simulink library "ET3036TU_model_library_2021b"  (R2021b)
settings: Solver=VariableStepAuto  StartTime=0.0  StopTime=10.0  RelTol=1e-3
values from neighbouring files (symbols this model uses):
  Data =     [Data.mat]
  E_tol = 100    [run_test.m]
  Fnom = 50    [run_test.m]
  OverChargingProtection = 0    [run_test.m]
  simulation_mode = 2    [run_test.m]
  T_err = 60*60    (= 3600)    [run_test.m]
  Tsample = 60    [run_test.m]
  Vnom = sqrt(3)*230    [run_test.m]
undefined symbols (not defined in the file or in its folder): sigbuilder_block, sim_text
libraries: simulink x13, spsThreePhaseDynamicLoadLib x5, spsPower3phPhasorLib x3, eePowerMeasurement x2, spsThreePhaseVIMeasurementLib x2, spsThreePhaseSourceLib x2, spspowerguiLib x2, spsPower3phInstantaneousLib x1, spsThreePhaseSeriesRLCLoadLib x1, $bdroot x1
(part 2 of 2)

== system ET3036TU_model_library_2021b/Energy Storage/Battery over charging// discharging Protection/Under Charging Protection ==
  SOC (%) : Inport
  Pref : Inport  Port=2
  Constant1 : Constant  Value=ovrchargpro
  Constant2 : Constant  Value=LowChrgLim
  GreaterThan : RelationalOperator  Operator=<=  OutDataTypeStr=boolean  RndMeth=Simplest
  GreaterThan1 : RelationalOperator  Operator=>  OutDataTypeStr=boolean  RndMeth=Simplest
  Logical Operator : Logic  AllPortsSameDT=off  OutDataTypeStr=boolean
  MATLAB Function : MATLAB Function  TreatAsAtomicUnit=on
  Switch : Switch  Criteria=u2 ~= 0
  Zero : Constant  Value=0  OutDataTypeStr=Inherit: Inherit via back propagation
  Zero1 : Constant  Value=0  OutDataTypeStr=Inherit: Inherit via back propagation
  wires:
  Logical Operator/1 -> Switch/1
  Zero1/1 -> Switch/3
  Constant1/1 -> Switch/2
  Switch/1 -> MATLAB Function/1(u)
  Pref/1 -> GreaterThan1/1
  GreaterThan/1 -> Logical Operator/1
  Constant2/1 -> GreaterThan/2
  GreaterThan1/1 -> Logical Operator/2
  Zero/1 -> GreaterThan1/2
  SOC (%)/1 -> GreaterThan/1

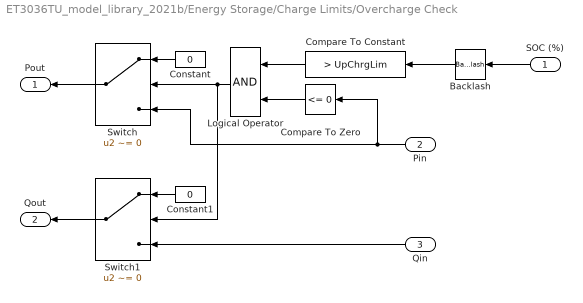
== system ET3036TU_model_library_2021b/Energy Storage/Charge Limits/Overcharge Check ==
  SOC (%) : Inport
  Pin : Inport  Port=2
  Qin : Inport  Port=3
  Backlash : Backlash  BacklashWidth=1e-3  InitialOutput=Initial_kWh_pc  ZeroCross=off
  Compare To Constant : simulink/Logic and Bit Operations/Compare To Constant  relop=>  const=UpChrgLim  OutDataTypeStr=boolean
  Compare To Zero : simulink/Logic and Bit Operations/Compare To Zero  relop=<=  OutDataTypeStr=boolean
  Constant : Constant  Value=0
  Constant1 : Constant  Value=0
  Logical Operator : Logic  AllPortsSameDT=off  OutDataTypeStr=boolean
  Switch : Switch  Criteria=u2 ~= 0
  Switch1 : Switch  Criteria=u2 ~= 0
  Pout : Outport  VectorParamsAs1DForOutWhenUnconnected=off
  Qout : Outport  Port=2  VectorParamsAs1DForOutWhenUnconnected=off
  wires:
  Backlash/1 -> Compare To Constant/1
  Switch1/1 -> Qout/1
  Constant1/1 -> Switch1/1
  Qin/1 -> Switch1/3
  Compare To Zero/1 -> Logical Operator/2
  Switch/1 -> Pout/1
  Pin/1 -> Switch/3, Compare To Zero/1
  SOC (%)/1 -> Backlash/1
  Constant/1 -> Switch/1
  Logical Operator/1 -> Switch/2, Switch1/2
  Compare To Constant/1 -> Logical Operator/1

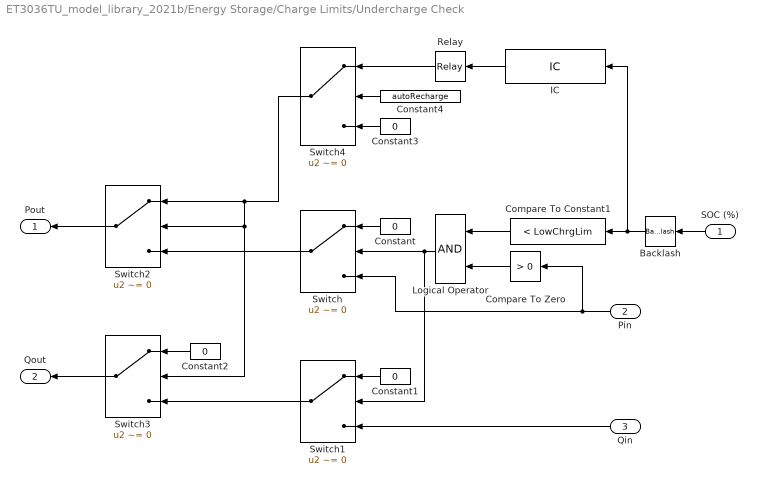
== system ET3036TU_model_library_2021b/Energy Storage/Charge Limits/Undercharge Check ==
  SOC (%) : Inport
  Pin : Inport  Port=2
  Qin : Inport  Port=3
  Backlash : Backlash  BacklashWidth=1e-3  InitialOutput=Initial_kWh_pc  ZeroCross=off
  Compare To Constant1 : simulink/Logic and Bit Operations/Compare To Constant  relop=<  const=LowChrgLim  OutDataTypeStr=boolean
  Compare To Zero : simulink/Logic and Bit Operations/Compare To Zero  relop=>  OutDataTypeStr=boolean
  Constant{,1..3} (4 alike) : Constant  Value=0
  Constant4 : Constant  Value=autoRecharge
  IC : InitialCondition  Value=RechargeSOC
  Logical Operator : Logic  AllPortsSameDT=off  OutDataTypeStr=boolean
  Relay : Relay  OnSwitchValue=RechargeSOC  OffSwitchValue=LowChrgLim  OnOutputValue=0  OffOutputValue=-Precharge/100*Pnom
  Switch{,1..4} (5 alike) : Switch  Criteria=u2 ~= 0
  Pout : Outport  VectorParamsAs1DForOutWhenUnconnected=off
  Qout : Outport  Port=2  VectorParamsAs1DForOutWhenUnconnected=off
  wires:
  Constant4/1 -> Switch4/2
  Constant3/1 -> Switch4/3
  Relay/1 -> Switch4/1
  Constant2/1 -> Switch3/1
  Switch1/1 -> Switch3/3
  Switch3/1 -> Qout/1
  Switch2/1 -> Pout/1
  Switch/1 -> Switch2/3
  IC/1 -> Relay/1
  Switch4/1 -> Switch3/2, Switch2/2, Switch2/1
  Backlash/1 -> Compare To Constant1/1, IC/1
  Qin/1 -> Switch1/3
  Constant1/1 -> Switch1/1
  Compare To Constant1/1 -> Logical Operator/1
  Logical Operator/1 -> Switch1/2, Switch/2
  Constant/1 -> Switch/1
  SOC (%)/1 -> Backlash/1
  Pin/1 -> Compare To Zero/1, Switch/3
  Compare To Zero/1 -> Logical Operator/2

== system ET3036TU_model_library_2021b/Voltage//frequency regulator/Bus Meassurement /Power Meassurement ==
  note: 1) Add Subsystem or Model blocks as valid variant choices.
      | 2) You cannot connect blocks at this level. At simulation, connectivity is automatically
      | determined, based on the active variant and port name matching.
  V : Inport
  I : Inport  Port=2
  discrete : Subsystem  VariantControl=simulation_mode==1
  phasor : Subsystem  VariantControl=simulation_mode==2
  P : Outport
  Q : Outport  Port=2

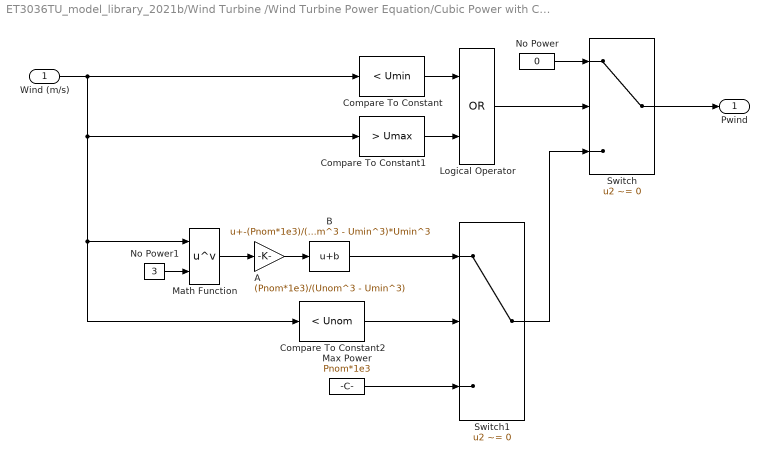
== system ET3036TU_model_library_2021b/Wind Turbine /Wind Turbine Power Equation/Cubic Power with Cutoff ==
  Wind (m/s) : Inport
  A : Gain  Gain=(Pnom*1e3)/(Unom^3 - Umin^3)
  B : Bias  Bias=-(Pnom*1e3)/(Unom^3 - Umin^3)*Umin^3
  Compare To Constant : simulink/Logic and Bit Operations/Compare To Constant  relop=<  const=Umin  OutDataTypeStr=boolean
  Compare To Constant1 : simulink/Logic and Bit Operations/Compare To Constant  relop=>  const=Umax  OutDataTypeStr=boolean
  Compare To Constant2 : simulink/Logic and Bit Operations/Compare To Constant  relop=<  const=Unom  OutDataTypeStr=boolean
  Logical Operator : Logic  Operator=OR  AllPortsSameDT=off  OutDataTypeStr=boolean
  Math Function : Math  Operator=pow  SignedPower=on  SaturateOnIntegerOverflow=on
  Max Power : Constant  Value=Pnom*1e3
  No Power : Constant  Value=0
  No Power1 : Constant  Value=3
  Switch : Switch  Criteria=u2 ~= 0  ZeroCross=off
  Switch1 : Switch  Criteria=u2 ~= 0  ZeroCross=off
  Pwind : Outport  VectorParamsAs1DForOutWhenUnconnected=off
  wires:
  B/1 -> Switch1/1
  Compare To Constant2/1 -> Switch1/2
  Compare To Constant1/1 -> Logical Operator/2
  Math Function/1 -> A/1
  No Power1/1 -> Math Function/2
  No Power/1 -> Switch/1
  Switch1/1 -> Switch/3
  Max Power/1 -> Switch1/3
  Wind (m/s)/1 -> Compare To Constant/1, Compare To Constant1/1, Math Function/1, Compare To Constant2/1
  A/1 -> B/1
  Logical Operator/1 -> Switch/2
  Switch/1 -> Pwind/1
  Compare To Constant/1 -> Logical Operator/1

== system ET3036TU_model_library_2021b/Wind Turbine /Wind Turbine Power Equation/Wind Turbine Properties ==
  Wind (m/s) : Inport
  Compare To Constant : simulink/Logic and Bit Operations/Compare To Constant  relop=<  const=Umin  OutDataTypeStr=boolean
  Compare To Constant1 : simulink/Logic and Bit Operations/Compare To Constant  relop=>  const=Umax  OutDataTypeStr=boolean
  Compare To Constant2 : simulink/Logic and Bit Operations/Compare To Constant  relop=<  const=Unom  OutDataTypeStr=boolean
  Logical Operator : Logic  Operator=OR  AllPortsSameDT=off  OutDataTypeStr=boolean
  Max Power : Constant  Value=Pnom*1e3
  No Power : Constant  Value=0
  Properties : Subsystem
  Switch : Switch  Criteria=u2 ~= 0  ZeroCross=off
  Switch1 : Switch  Criteria=u2 ~= 0  ZeroCross=off
  Pwind : Outport  VectorParamsAs1DForOutWhenUnconnected=off
  wires:
  Compare To Constant/1 -> Logical Operator/1
  Switch/1 -> Pwind/1
  Logical Operator/1 -> Switch/2
  Wind (m/s)/1 -> Compare To Constant2/1, Properties/1(In1), Compare To Constant1/1, Compare To Constant/1
  Max Power/1 -> Switch1/3
  Switch1/1 -> Switch/3
  No Power/1 -> Switch/1
  Compare To Constant1/1 -> Logical Operator/2
  Compare To Constant2/1 -> Switch1/2
  Properties/1(Out1) -> Switch1/1

== system ET3036TU_model_library_2021b/Voltage//frequency regulator/Bus Meassurement /Power Meassurement/discrete ==
  V : Inport
  I : Inport  Port=2
  Power Measurement (Three-Phase) : eePowerMeasurement/Power Measurement (Three-Phase)  LabelModeActiveChoice=Discrete  F=Fnom  K=1  Seq=Positive  Ts=Tsample
      settings: SourceProductBaseCode=PS
  P : Outport
  Q : Outport  Port=2
  wires:
  V/1 -> Power Measurement (Three-Phase)/1
  I/1 -> Power Measurement (Three-Phase)/2
  Power Measurement (Three-Phase)/1 -> P/1
  Power Measurement (Three-Phase)/2 -> Q/1

== system ET3036TU_model_library_2021b/Voltage//frequency regulator/Bus Meassurement /Power Meassurement/phasor ==
  V : Inport
  I : Inport  Port=2
  "Power (3ph, Phasor)" : spsPower3phPhasorLib/Power (3ph, Phasor)
      settings: SourceProductBaseCode=PS
  P : Outport
  Q : Outport  Port=2
  wires:
  V/1 -> "Power (3ph, Phasor)"/1
  I/1 -> "Power (3ph, Phasor)"/2
  "Power (3ph, Phasor)"/1 -> P/1
  "Power (3ph, Phasor)"/2 -> Q/1

== system ET3036TU_model_library_2021b/Wind Turbine /Wind Turbine Power Equation/Wind Turbine Properties/Properties ==
  In1 : Inport
  Air Density : Gain  Gain=rho
  Blade Swept Area (m^2) : Gain  Gain=A
  Gain : Gain  Gain=1/2
  Power Coefficient : Constant  Value=Cp
  "Product " : Product  SaturateOnIntegerOverflow=on  OutDataTypeStr=Inherit: Same as first input
  wind_speed^3 : Fcn  Expr=u(1)^3
  Out1 : Outport  VectorParamsAs1DForOutWhenUnconnected=off
  wires:
  Gain/1 -> Blade Swept Area (m^2)/1
  "Product "/1 -> Out1/1
  Air Density/1 -> Gain/1
  In1/1 -> wind_speed^3/1
  Power Coefficient/1 -> "Product "/2
  wind_speed^3/1 -> Air Density/1
  Blade Swept Area (m^2)/1 -> "Product "/1

== matlab function ET3036TU_model_library_2021b/MATLAB Function ==
  data: in1 input; out1 output; in2 input; out2 output
function [out1,out2] = Controller(in1,in2)
% An example function that takes two inputs (in1,in2) and gives two output
% (out1,out2)
out1 = in1;
out2 = in2;

== matlab function ET3036TU_model_library_2021b/Energy Storage/Battery over charging// discharging Protection/Over Charging Protection/MATLAB Function ==
  data: u input
function fcn(u)
    if u == 1
        error('Battery is fully charged (Max SOC% reached), hence cannot charge more. Increase SOC% or Check Pref signal')
    end

== matlab function ET3036TU_model_library_2021b/Energy Storage/Battery over charging// discharging Protection/Under Charging Protection/MATLAB Function ==
  data: u input
function fcn(u)
    if u == 1
        error('Battery is discharged fully (Min SOC% reached), hence cannot discharge more. Decrease SOC% or Check Pref signal')
    end

== matlab function ET3036TU_model_library_2021b/Energy Storage/Pref Limit Check/Simulation Stop ==
  data: u input
function  fcn(u)
if u<0
    error('Power reference to the battery exceeds the battery''s nominal power')
end

== matlab function ET3036TU_model_library_2021b/Diesel generator/Simulation interruptor ==
  data: u input
function  fcn(u)
if u<0
    error('-ve reference given to disele generator. Disele generator cannot absorb power. ')
end

== matlab function ET3036TU_model_library_2021b/Voltage//frequency regulator/Simulation interruptor ==
  data: u input
function  fcn(u)
if u==1
    error('Simulation interrupted: System supply/demand imbalance.')
end
